simulink model "wind_turbine_control_basic_model"  (R2018a)
settings: Solver=VariableStepAuto  StartTime=0.0  StopTime=10.0  RelTol=1e-3
libraries: re_lib x1
settings Model: Creator=chaka  LastModifiedBy=chaka

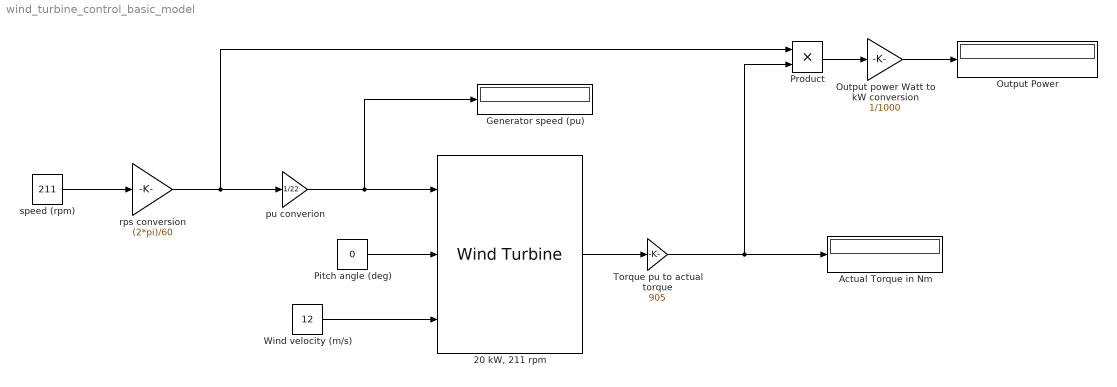
== system wind_turbine_control_basic_model ==
  "20 kW, 211 rpm" : re_lib/Wind Generation/Wind Turbine  Pnom=20e3  Pelec_base=20e3/0.9  wind_base=12  P_wind_base=1  speed_nom=1  pitch_angle=0  c1_c6="[0.51763          116          0.4            5           21     0.006795]"  cp_nom=0.48  lambda_nom=8.1
      settings: SourceProductName=Simscape Power Systems  SourceProductBaseCode=PS
  Actual Torque in Nm : Display
  Generator speed (pu) : Display
  Output Power : Display
  Output power Watt to kW conversion : Gain  Gain=1/1000
  Pitch angle (deg) : Constant  Value=0
  Product : Product
  "Torque pu to actual torque " : Gain  Gain=905
  Wind velocity (m/s) : Constant  Value=12
  pu converion : Gain  Gain=1/22
  rps conversion : Gain  Gain=(2*pi)/60
  speed (rpm) : Constant  Value=211
  wires:
  speed (rpm)/1 -> rps conversion/1
  rps conversion/1 -> Product/1, pu converion/1
  pu converion/1 -> "20 kW, 211 rpm"/1, Generator speed (pu)/1
  "20 kW, 211 rpm"/1 -> "Torque pu to actual torque "/1
  Wind velocity (m/s)/1 -> "20 kW, 211 rpm"/3
  Pitch angle (deg)/1 -> "20 kW, 211 rpm"/2
  "Torque pu to actual torque "/1 -> Product/2, Actual Torque in Nm/1
  Product/1 -> Output power Watt to kW conversion/1
  Output power Watt to kW conversion/1 -> Output Power/1
